simulink model "c9mdde1b"  (R2022a)
settings: Solver=VariableStepAuto  StartTime=0.0  StopTime=10.0  RelTol=1e-3
settings Model: Creator=xuedi  LastModifiedBy=xuedi

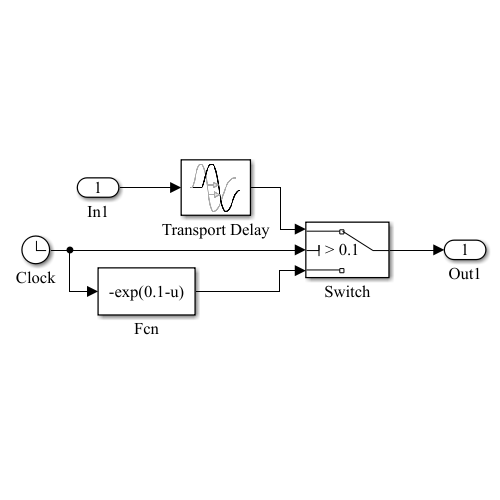
[thumbnail: Simulink's stored preview of the top-level diagram]
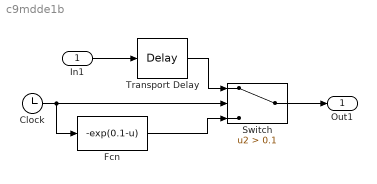
== system c9mdde1b ==
  In1 : Inport
  Clock : Clock
  Fcn : Fcn  Expr=-exp(0.1-u)
  Switch : Switch  Criteria=u2 > Threshold  Threshold=0.1  SaturateOnIntegerOverflow=off  InputSameDT=off
  Transport Delay : TransportDelay
  Out1 : Outport
  wires:
  In1/1 -> Transport Delay/1
  Clock/1 -> Fcn/1, Switch/2
  Fcn/1 -> Switch/3
  Switch/1 -> Out1/1
  Transport Delay/1 -> Switch/1
